simulink model "Lab3_test"  (R2017a)
settings: Solver=ode3  StartTime=0.0  StopTime=0.004  FixedStep=2e-6  RelTol=1e-5  EnableMultiTasking=on
libraries: commfilt2 x2, commchan3 x1, commsink2 x1, commrandsrc2 x1
settings Model: Creator=Dennis Silage  LastModifiedBy=chris
settings DataIOCC: LimitDataPoints=on  SaveFormat=Array  SignalLoggingSaveFormat=ModelDataLogs
settings OptimizationCC: ExpressionDepthLimit=2147483647  InitFltsAndDblsToZero=on  LifeSpan=inf
settings DebuggingCC: UnderspecifiedInitializationDetection=Classic  MergeDetectMultiDrivingBlocksExec=none  FcnCallInpInsideContextMsg=warning  StateNameClashWarn=warning  SFUnexpectedBacktrackingDiag=warning  SFNoUnconditionalDefaultTransitionDiag=warning  SFExecutionAtInitializationDiag=none
settings HardwareCC: ProdBitPerPointer=32  ProdBitPerSizeT=32  ProdBitPerPtrDiffT=32  ProdLargestAtomicFloat=None  ProdIntDivRoundTo=Undefined  ProdEndianess=Unspecified  ProdWordSize=32  ProdHWDeviceType=32-bit Generic
settings ModelReferenceCC: PropagateSignalLabelsOutOfModel=off
settings GRTTargetCC: TargetLangStandard=C89/C90 (ANSI)  GeneratePreprocessorConditionals=Disable all  CombineOutputUpdateFcns=off  GRTInterface=on
settings ConfigComp: CovMetricSettings=dw  CovHtmlReporting=on  CovSaveCumulativeToWorkspaceVar=on  CovSaveSingleToWorkspaceVar=on  CovExternalEMLEnable=off  CovSFcnEnable=off

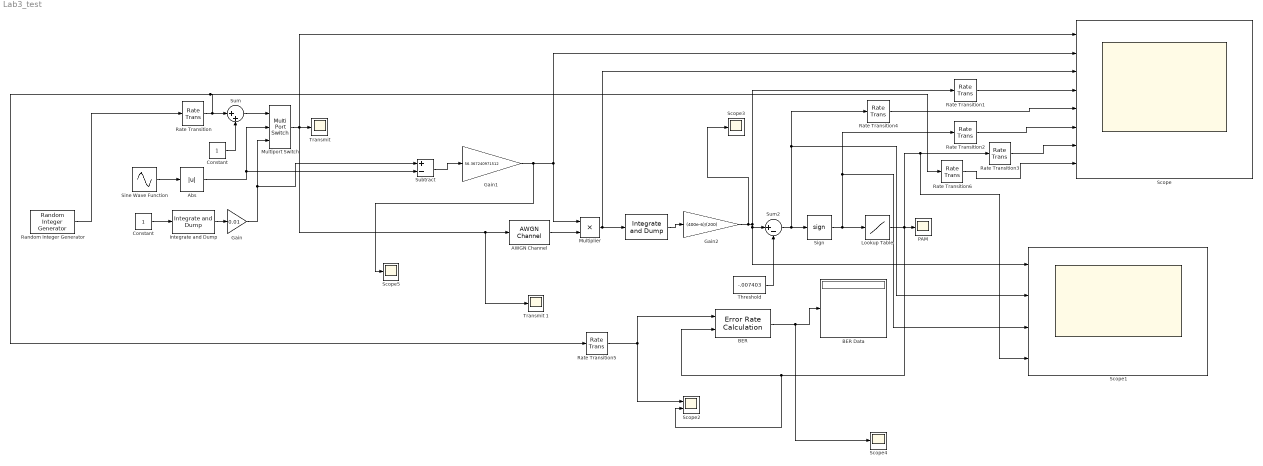
== system Lab3_test ==
  " " : commfilt2/Integrate and Dump  obssamples=200  offsetsamples=0  nodump=off  roundingMode=Floor  overflowMode=on  outputDataTypeStr=Inherit: Same as accumulator  outputLastDataTypeStr=Inherit: Same as accumulator
      settings: SourceProductName=Communications System Toolbox
  AWGN Channel : commchan3/AWGN Channel  InputProcessing=Inherited (this choice will be removed - see release notes)  seed=randseed  noiseMode=Variance from mask  EbNodB=40  EsNodB=10  SNRdB=10  bitsPerSym=1  Ps=25  Tsym=400e-6  variance=0
  Abs : Abs
  BER : commsink2/Error Rate Calculation  N=1  st_delay=0  cp_mode=Entire frame  subframe=[]  PMode=Port  WsName=ErrorVec  RsMode2=off  stop=off  numErr=100  maxBits=1e6
  BER Data : Display
  Constant : Constant
  "Constant " : Constant  SampleTime=2e-6
  Gain : Gain  Gain=0.01
  Gain1 : Gain  Gain=56.367240971512
  Gain2 : Gain  Gain=(400e-6)/(200)
  Integrate and Dump : commfilt2/Integrate and Dump  obssamples=200  offsetsamples=0  nodump=on  roundingMode=Floor  overflowMode=off  outputDataTypeStr=Inherit: Same as accumulator  outputLastDataTypeStr=Inherit: Same as accumulator
      settings: SourceProductName=Communications System Toolbox
  Lookup Table : Lookup_n-D  NumberOfTableDimensions=1  BreakpointsForDimension1=[-1, 0,1]  Table=[0,0, 1]  InternalRulePriority=Speed  RndMeth=Nearest  InputSameDT=on
  Multiplier : Product  RndMeth=Zero
  Multiport Switch : MultiPortSwitch  Inputs=2
  "PAM " : Scope
  Random Integer Generator : commrandsrc2/Random Integer Generator  mul=2  seed=randseed  Ts=400e-6  frameBased=off  sampPerFrame=50  orient=on  outDataType=double
  Rate Transition{,1..4,6} (6 alike) : RateTransition
  Rate Transition5 : RateTransition  OutPortSampleTime=400e-6
  Scope : Scope  NumInputPorts=8
  Scope1 : Scope  NumInputPorts=4
  Scope2 : Scope  NumInputPorts=2
  Scope3 : Scope
  Scope4 : Scope
  Scope5 : Scope
  Sign : Signum
  Sine Wave Function : Sin  SineType=Sample based  Amplitude=2  Frequency=2*pi*0.0005  Samples=400  SampleTime=2e-6
  Subtract : Sum  Inputs=+-
  Sum : Sum  Inputs=|++
  Sum2 : Sum  Inputs=|+-
  Threshold : Constant  Value=-.007403
  Transmit : Scope
  Transmit 1 : Scope
  wires:
  Rate Transition/1 -> Rate Transition6/1, Rate Transition5/1, Sum/1
  Sum/1 -> Multiport Switch/1
  Constant/1 -> Sum/2
  Integrate and Dump/1 -> Gain/1
  "Constant "/1 -> Integrate and Dump/1
  Sine Wave Function/1 -> Abs/1
  Abs/1 -> Subtract/2, Multiport Switch/2
  Subtract/1 -> Gain1/1
  Gain/1 -> Subtract/1, Multiport Switch/3
  Multiport Switch/1 -> Scope/1, Transmit 1/1, AWGN Channel/1, Transmit/1
  AWGN Channel/1 -> Multiplier/2
  BER/1 -> Scope4/1, BER Data/1
  Sum2/1 -> Scope1/2, Rate Transition4/1, Sign/1
  Lookup Table/1 -> Scope1/4, Rate Transition3/1, "PAM "/1, Scope2/2, BER/2
  Random Integer Generator/1 -> Rate Transition/1
  Threshold/1 -> Sum2/2
  Sign/1 -> Scope1/3, Rate Transition2/1, Lookup Table/1
  Gain1/1 -> Scope5/1, Multiplier/1, Scope/2
  Rate Transition1/1 -> Scope/4
  Rate Transition2/1 -> Scope/6
  Rate Transition3/1 -> Scope/7
  Rate Transition4/1 -> Scope/5
  Multiplier/1 -> " "/1, Scope/3
  " "/1 -> Gain2/1
  Rate Transition5/1 -> BER/1, Scope2/1
  Rate Transition6/1 -> Scope/8
  Gain2/1 -> Scope3/1, Scope1/1, Sum2/1, Rate Transition1/1
